simulink model "ExercitiiPlatforma"  (R2016a)
settings: Solver=VariableStepDiscrete  StartTime=0.0  StopTime=600  RelTol=1e-3
undefined symbols (not defined in the file): m, n
settings Model: Creator=Cristina  LastModifiedBy=Cristina

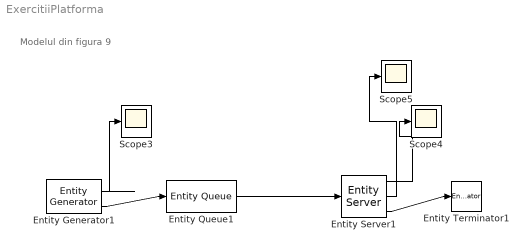
== system ExercitiiPlatforma ==
  note: Modelul din figura 9
  Entity Generator1 : EntityGenerator  OutputPortMessageModes=n,m  TimeSource=MATLAB action  IntergenerationTimeAction=|  GenerateAction=|  AttributeName=ServiceTime  AttributeInitialValue=32  NumberEntitiesDeparted=on  EntityType=Structured  EntityTypeName=Entity
      IntergenerationTimeAction=|
      | persistent init
      | if (isempty(init))
      |     rng(236);
      |     init = true;
      | end
      | dt= 12 + rand * 12;
      GenerateAction=|
      | persistent st
      | if (isempty(st))
      |     rng(462);
      |     st = true;
      | end
      | entity.ServiceTime = 28 + 8 * rand;
      settings: OutputPortMap=o0,o3
  Entity Queue1 : EntityQueue  InputPortMessageModes=m  OutputPortMessageModes=m
      settings: OutputPortMap=o5
  Entity Server1 : EntityServer  InputPortMessageModes=m  OutputPortMessageModes=n,n,m  Capacity=2  ServiceTimeSource=Attribute  ServiceTimeAction=|  NumberEntitiesDeparted=on  AverageWait=on
      | persistent init
      | if (isempty(init))
      |     rng(123);
      |     init = true;
      | end
      | dt = 28 + 12 * rand
      settings: OutputPortMap=o0,o4,o9
  Entity Terminator1 : EntityTerminator  InputPortMessageModes=m
  Scope3 : Scope
  Scope4 : Scope
  Scope5 : Scope
  wires:
  Entity Server1/3 -> Entity Terminator1/1
  Entity Generator1/2 -> Entity Queue1/1
  Entity Queue1/1 -> Entity Server1/1
  Entity Generator1/1 -> Scope3/1
  Entity Server1/1 -> Scope4/1
  Entity Server1/2 -> Scope5/1
